simulink model "Power_Subsystem_Designer"  (R2022b)
settings: Solver=VariableStepAuto  StartTime=0.0  StopTime=1  MaxStep=0.0001  RelTol=1e-3
values from neighbouring files (symbols this model uses):
  motorControllerCurve = [25, 260 ... (first row only)    [crayon_box.m]
  motorTempCurve = (1 - motorCoef *      (motorTempX / maxMotorTemp) .^ 2)    [blue_crayon.m]    (also in crayon_box.m = 140 -  (motorTempX - minMotorTemp) .^ 2 .* (140) / (maxMotor)
  motorTempX = 0 : maxMotorTemp / STEP_SIZE : maxMotorTemp    [blue_crayon.m]    (also in crayon_box.m = minMotorTemp : (maxMotorTemp-minMotorTemp) / STEPS : maxMoto)
  throttleCurve = polyval([1 0], throttleX)    [crayon_box.m]
  throttleX = 0:1/STEPS:1    [crayon_box.m]
libraries: simulink x1
settings Model: Creator=Inver  LastModifiedBy=dagge
settings ModelReferenceCC: EnableRefExpFcnMdlSchedulingChecks=on

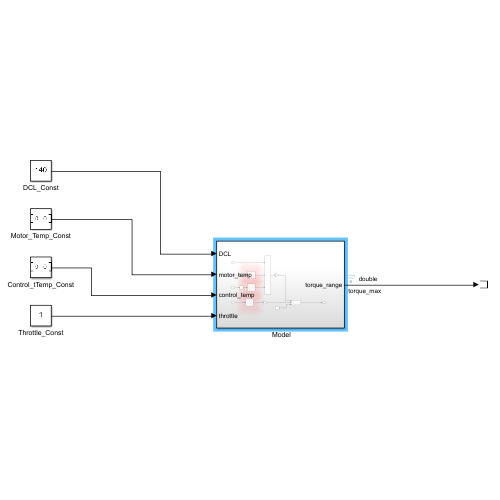
[thumbnail: Simulink's stored preview of the top-level diagram]
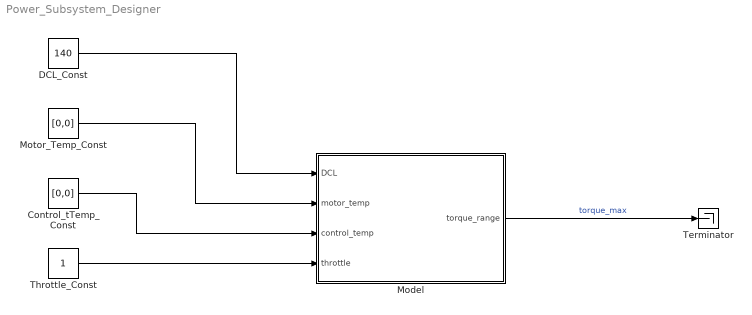
== system Power_Subsystem_Designer ==
  " Model" : Subsystem
  Control_tTemp_Const : Constant  Value=[0,0]
  DCL_Const : Constant  Value=140  SampleTime=10
  Motor_Temp_Const : Constant  Value=[0,0]
  Terminator : Terminator
  Throttle_Const : Constant
  wires:
  " Model"/1(torque_range) -> Terminator/1  "torque_max"
  DCL_Const/1 -> " Model"/1(DCL)
  Control_tTemp_Const/1 -> " Model"/3(control_temp)
  Motor_Temp_Const/1 -> " Model"/2(motor_temp)
  Throttle_Const/1 -> " Model"/4(throttle)

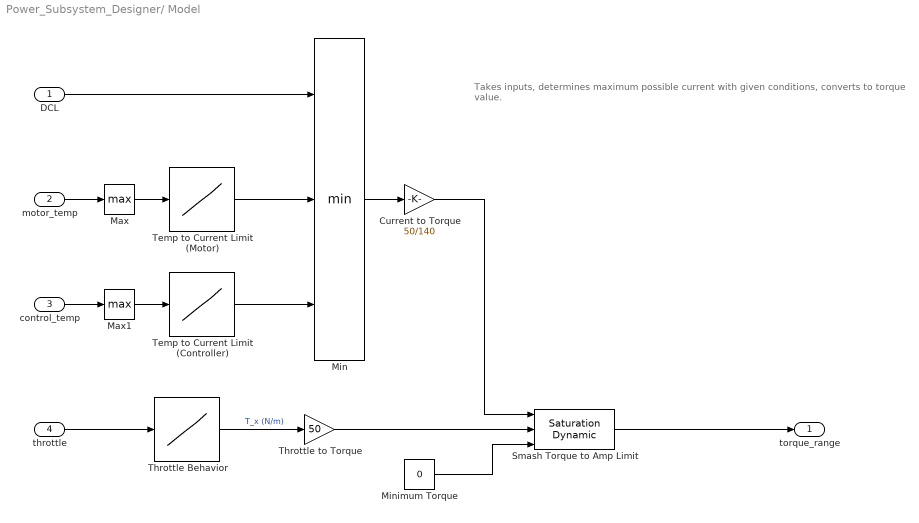
== system Power_Subsystem_Designer/ Model ==
  note: Takes inputs, determines maximum possible current with given conditions, converts to torque value.
  DCL : Inport
  motor_temp : Inport  Port=2
  control_temp : Inport  Port=3
  throttle : Inport  Port=4
  Current to Torque : Gain  Gain=50/140
  Max : MinMax  Function=max
  Max1 : MinMax  Function=max
  Min : MinMax  Inputs=3
  "Minimum Torque " : Constant  Value=0
  Smash Torque to Amp Limit : simulink/Discontinuities/Saturation Dynamic  OutMin=[0]  OutMax=[]  OutDataTypeStr=Inherit: Same as second input  OutDataType=fixdt(1, 16)  OutScaling=2^-10  DoSatur=off
  Temp to Current Limit (Controller) : Lookup_n-D  NumberOfTableDimensions=1  BreakpointsForDimension1=motorControllerCurve(:,1)  IndexSearchMethod=Evenly spaced points  Table=motorControllerCurve(:,2)  ExtrapMethod=Clip  UseLastTableValue=on  InternalRulePriority=Speed  RndMeth=Simplest
  Temp to Current Limit (Motor) : Lookup_n-D  NumberOfTableDimensions=1  BreakpointsForDimension1=motorTempX  IndexSearchMethod=Evenly spaced points  Table=motorTempCurve  ExtrapMethod=Clip  UseLastTableValue=on  InternalRulePriority=Speed  RndMeth=Simplest
  "Throttle Behavior " : Lookup_n-D  NumberOfTableDimensions=1  BreakpointsForDimension1=throttleX  IndexSearchMethod=Evenly spaced points  Table=throttleCurve  InternalRulePriority=Speed  RndMeth=Simplest
  Throttle to Torque : Gain  Gain=50
  torque_range : Outport  OutDataTypeStr=double  LockScale=on
  wires:
  motor_temp/1 -> Max/1
  Max/1 -> Temp to Current Limit (Motor)/1
  control_temp/1 -> Max1/1
  Temp to Current Limit (Controller)/1 -> Min/3
  Temp to Current Limit (Motor)/1 -> Min/2
  DCL/1 -> Min/1
  Min/1 -> Current to Torque/1
  "Minimum Torque "/1 -> Smash Torque to Amp Limit/3
  Smash Torque to Amp Limit/1 -> torque_range/1
  throttle/1 -> "Throttle Behavior "/1
  "Throttle Behavior "/1 -> Throttle to Torque/1  "T_x (N/m)"
  Throttle to Torque/1 -> Smash Torque to Amp Limit/2
  Current to Torque/1 -> Smash Torque to Amp Limit/1
  Max1/1 -> Temp to Current Limit (Controller)/1
